simulink model "pam_ser_v9_fixed"  (R2024b)
settings: Solver=FixedStepDiscrete  StartTime=0.0  StopTime=num_symbols  RelTol=1e-3
InitFcn:
  | if ~exist('M','var'), M=4; end; if ~exist('osr','var'), osr=8; end; if ~exist('rolloff','var'), rolloff=0.5; end; if ~exist('span','var'), span=6; end; if ~exist('num_symbols','var'), num_symbols=1e5; end; if ~exist('EbN0dB','var'), EbN0dB=10; end; k = log2(M); Es = 1; Eb = Es/k; snr_lin = 10^(EbN0dB/10); N0 = Eb / snr_lin; NoiseVar = (N0/2)*osr; RRC_Delay = span; Rect_Delay = 1;
values from neighbouring files (symbols this model uses):
  M = M_values(m_idx)    [SER_PAM_code.m]
  osr = 8    [SER_PAM_code.m]
  rolloff = 0.5    [SER_PAM_code.m]
  span = 6    [SER_PAM_code.m]
libraries: commfilt2 x4, commdigbbndam3 x3, commchan3 x2, commsink2 x2, commrandsrc3 x1, dspsigops x1
settings Model: Creator=abdel  LastModifiedBy=abdel

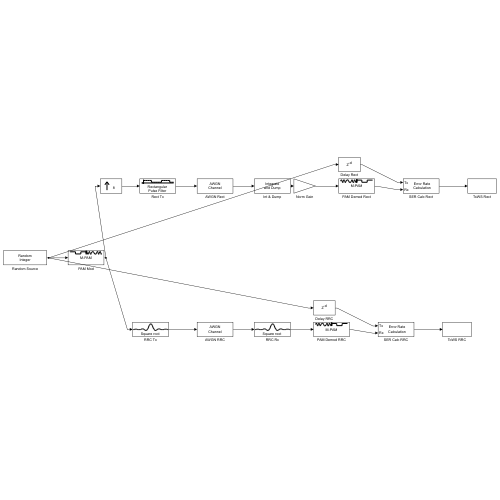
[thumbnail: Simulink's stored preview of the top-level diagram]
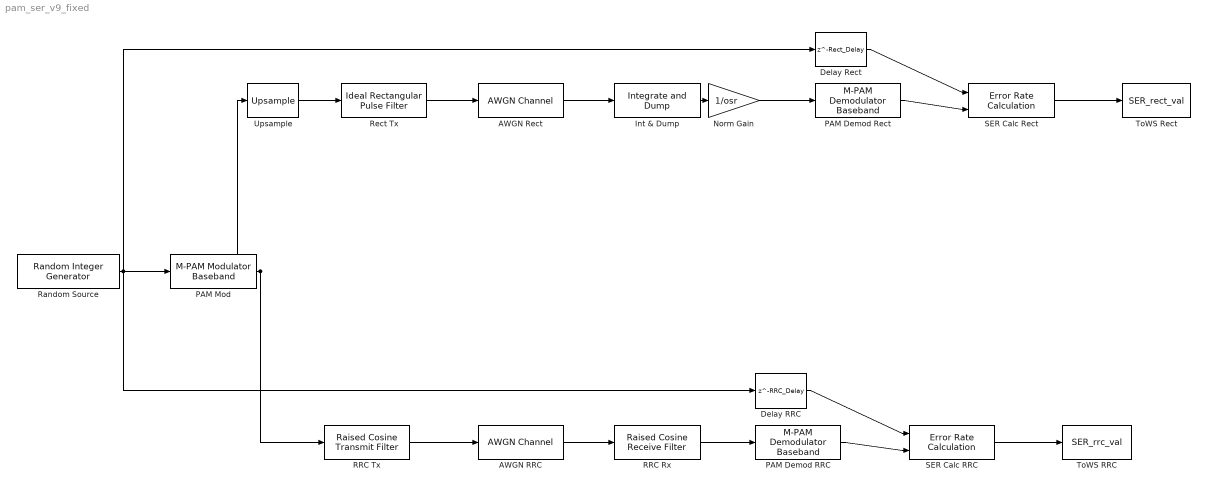
== system pam_ser_v9_fixed ==
  AWGN RRC : commchan3/AWGN Channel  LegacyMode=off  NoiseMethod=Variance  noiseMode="Signal to noise ratio  (SNR)"  EbNo=10  EsNo=10  SNR=10  BitsPerSymbol=1  SignalPower=1  SamplesPerSymbol=1  SymbolPeriod=1  VarianceSource=Parameter  Variance=NoiseVar  RandomStream=Global stream  Seed=67  SimulateUsing=Code generation
  AWGN Rect : commchan3/AWGN Channel  LegacyMode=off  NoiseMethod=Variance  noiseMode="Signal to noise ratio  (SNR)"  EbNo=10  EsNo=10  SNR=10  BitsPerSymbol=1  SignalPower=1  SamplesPerSymbol=1  SymbolPeriod=1  VarianceSource=Parameter  Variance=NoiseVar  RandomStream=Global stream  Seed=67  SimulateUsing=Code generation
  Delay RRC : Delay  DelayLength=RRC_Delay
  Delay Rect : Delay  DelayLength=Rect_Delay
  Int & Dump : commfilt2/Integrate and Dump  obssamples=osr  offsetsamples=0  nodump=off  roundingMode=Floor  overflowMode=off  outputDataTypeStr=Inherit: Same as accumulator  outputLastDataTypeStr=Inherit: Same as accumulator
  Norm Gain : Gain  Gain=1/osr
  PAM Demod RRC : commdigbbndam3/M-PAM Demodulator Baseband  M=M  OutType=Integer  Dec=Gray  PowType=Average Power  MinDist=2  AvgPow=1  PeakPow=1  outDtype1=Inherit via internal rule  outDtype2=Inherit via internal rule  denormFactorWordLen=16  denormFactorDataTypeStr=Inherit: Same word length as input  denormFactorLastDataTypeStr=Inherit: Same word length as input  prodOutWordLen=16  prodOutRoundingMode=Floor  prodOutOverflowMode=Wrap  prodOutOvFlMode=off  prodOutOvFlModeLastStrValue=off  sumWordLen=16
  PAM Demod Rect : commdigbbndam3/M-PAM Demodulator Baseband  M=M  OutType=Integer  Dec=Gray  PowType=Average Power  MinDist=2  AvgPow=1  PeakPow=1  outDtype1=Inherit via internal rule  outDtype2=Inherit via internal rule  denormFactorWordLen=16  denormFactorDataTypeStr=Inherit: Same word length as input  denormFactorLastDataTypeStr=Inherit: Same word length as input  prodOutWordLen=16  prodOutRoundingMode=Floor  prodOutOverflowMode=Wrap  prodOutOvFlMode=off  prodOutOvFlModeLastStrValue=off  sumWordLen=16
  PAM Mod : commdigbbndam3/M-PAM Modulator Baseband  M=M  InType=Integer  Enc=Gray  PowType=Average Power  MinDist=2  AvgPow=1  PeakPow=1  outDtype=double  outWordLen=16  outUDDataType=sfix(16)  outFracLenMode=Best precision  outFracLen=15  outDataTypeStr=double  outLastDataTypeStr=double
  RRC Rx : commfilt2/Raised Cosine Receive Filter  filtType=Square root  R=rolloff  filtSpan=span  N=osr  downFactor=osr  downOffset=0  filterGain=1  InputProcessing=Columns as channels (frame based)  RateOptions=Enforce single-rate processing  framing=Mute  checkCoeff=off  variableName=rcRxFilt  currentFiltSpan=10  D=5  inputOffset=0  sampMode=Mute  saveAsFlag=0  rateMode=Downsampling  checkGain=Normalized  launchFVT=on  roundingMode=Floor  overflowMode=off  coeffDataTypeStr=Inherit: Same word length as input  coeffMin=[]  coeffMax=[]  coeffLastDataTypeStr=Inherit: Same word length as input  accumDataTypeStr=Inherit: Same as product output  accumLastDataTypeStr=Inherit: Same as product output  outputDataTypeStr=Inherit: Same as accumulator  outputMin=[]  outputMax=[]  outputLastDataTypeStr=Inherit: Same as accumulator
  RRC Tx : commfilt2/Raised Cosine Transmit Filter  filtType=Square root  R=rolloff  filtSpan=span  N=osr  filterGain=1  InputProcessing=Columns as channels (frame based)  RateOptions=Enforce single-rate processing  framing=Mute  checkCoeff=off  variableName=rcTxFilt  checkGain=Normalized  sampMode=Mute  saveAsFlag=0  currentFiltSpan=10  D=(10)/2  launchFVT=on  roundingMode=Floor  overflowMode=off  coeffDataTypeStr=Inherit: Same word length as input  coeffMin=[]  coeffMax=[]  coeffLastDataTypeStr=Inherit: Same word length as input  outputDataTypeStr=Inherit: Same as accumulator  outputMin=[]  outputMax=[]  outputLastDataTypeStr=Inherit: Same as accumulator
  Random Source : commrandsrc3/Random Integer Generator  SetSize=M  SeedSource=Auto  Seed=0  SampleTime=1  SamplesPerFrame=1  OutputDataType=double  SimulateUsing=Interpreted execution
  Rect Tx : commfilt2/Ideal Rectangular Pulse Filter  pulseLen=osr  pulseDelay=0  InputProcessing=Columns as channels (frame based)  RateOptions=Enforce single-rate processing  sampMode=Mute  normCheck=off  normMode=Sum of samples  filterGain=1  saveAsFlag=0  roundingMode=Floor  overflowMode=off  firstCoeffDataTypeStr=Inherit: Same word length as input  firstCoeffMin=[]  firstCoeffMax=[]  firstCoeffLastDataTypeStr=Inherit: Same word length as input  outputDataTypeStr=Inherit: Same as accumulator  outputMin=[]  outputMax=[]  outputLastDataTypeStr=Inherit: Same as accumulator
  SER Calc RRC : commsink2/Error Rate Calculation  N=0  st_delay=0  cp_mode=Entire frame  subframe=[]  PMode=Port  WsName=ErrorVec  RsMode2=off  stop=off  numErr=100  maxBits=1e6
  SER Calc Rect : commsink2/Error Rate Calculation  N=0  st_delay=0  cp_mode=Entire frame  subframe=[]  PMode=Port  WsName=ErrorVec  RsMode2=off  stop=off  numErr=100  maxBits=1e6
  ToWS RRC : ToWorkspace  VariableName=SER_rrc_val  SampleTime=-1
  ToWS Rect : ToWorkspace  VariableName=SER_rect_val  SampleTime=-1
  Upsample : dspsigops/Upsample  FactorSource=Dialog parameter  N=osr  Nmax=16  phase=0  InputProcessing=Columns as channels (frame based)  RateOptions=Enforce single-rate processing  ic=0  mode=Unused parameter value
  wires:
  Random Source/1 -> PAM Mod/1, Delay Rect/1, Delay RRC/1
  PAM Mod/1 -> Upsample/1, RRC Tx/1
  Upsample/1 -> Rect Tx/1
  Rect Tx/1 -> AWGN Rect/1
  AWGN Rect/1 -> Int & Dump/1
  Int & Dump/1 -> Norm Gain/1
  Norm Gain/1 -> PAM Demod Rect/1
  Delay Rect/1 -> SER Calc Rect/1
  PAM Demod Rect/1 -> SER Calc Rect/2
  SER Calc Rect/1 -> ToWS Rect/1
  RRC Tx/1 -> AWGN RRC/1
  AWGN RRC/1 -> RRC Rx/1
  RRC Rx/1 -> PAM Demod RRC/1
  Delay RRC/1 -> SER Calc RRC/1
  PAM Demod RRC/1 -> SER Calc RRC/2
  SER Calc RRC/1 -> ToWS RRC/1
